simulink library "Fricciones"  (Simulink 8.3)
settings: Solver=ode45  StartTime=0.0  StopTime=10.0  RelTol=1e-3
undefined symbols (not defined in the file): Fc, Fc2, Fm, Friccion, Fs, Fs2, Fsc, mu_pts, Normal_Force_Pist_Cyl, To
libraries: nesl_utility x10, fl_lib x8, Fricciones x4, MS2G_SS_Intf_Lib x1
settings Model: Creator=Sebastian  LastModifiedBy=Sebastian

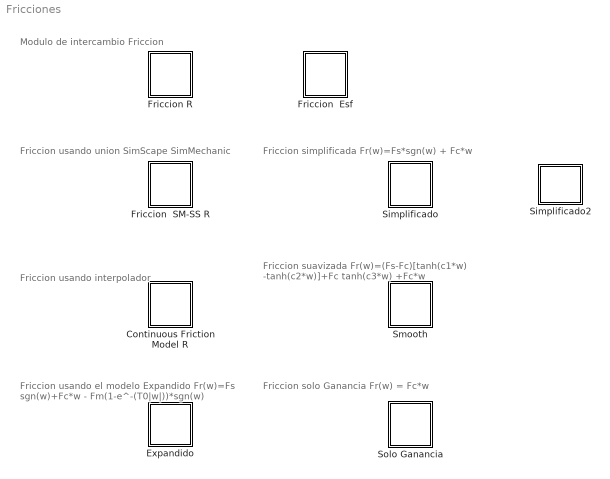
== system Fricciones ==
  note: Friccion usando
      | union SimScape
      | SimMechanic
  note: Modulo de
      | intercambio Friccion
  note: Friccion
      | simplificada
      |
      | Fr(w)=Fs*sgn(w) + Fc*w
  note: Friccion suavizada
      |
      | Fr(w)=(Fs-Fc)[tanh(c1*w)
      | -tanh(c2*w)]+Fc tanh(c3*w)
      | +Fc*w
  note: Friccion usando
      | el modelo
      | Expandido
      |
      | Fr(w)=Fs sgn(w)+Fc*w -
      | Fm(1-e^-(T0|w|))*sgn(w)
  note: Friccion solo
      | Ganancia
      |
      | Fr(w) = Fc*w
  note: Friccion usando
      | interpolador
  Continuous Friction Model R : Subsystem  mask{muk=Fc, mus=Fs, vth=0}
      mask init:
      | %%FRICTION CURVE
      | % Velocity vs. coefficient of friction
      | 
      | % NUMBER OF POINTS ON CURVE
      | num_fs_pts = 101;
      | 
      | % CURVE LIMITS
      | v_lowlim = -3*vth;
      | v_upplim = 3*vth;
      | 
      | % GENERATE X-AXIS POINTS (velocity)
      | v_pts = linspace(v_lowlim, v_upplim, num_fs_pts);
      | 
      | % DETERMINE Y-AXIS POINTS (coefficient of friction)
      | for i=1:num_fs_pts
      |     if(v_pts(i)<(-1.5*vth))
      |         mu_pts(i) = -muk;
      |     elseif(v_pts(i)>=-1.5*vth && v_pts(i)<-vth)
      |         mu_pts(i) = -(muk-mus)/(0.5*vth)*(-1.5*vth-v_pts(i))-muk;
      |     elseif(v_pts(i)>=-vth && v_pts(i)<vth)
      |         mu_pts(i) = -(mus)/vth*(-vth-v_pts(i))-mus;
      |     elseif(v_pts(i)>=vth && v_pts(i)<1.5*vth)
      |         mu_pts(i) = (muk-mus)/(0.5*vth)*(v_pts(i)-1.5*vth)+muk;
      |     elseif(v_pts(i)>=(1.5*vth))
      |         mu_pts(i) = muk;
      |     end
      | end
  Expandido : Subsystem
      mask init:
      | %To=0.1
      | %Fm=0.2
  Friccion  Esf : Subsystem
  Friccion  SM-SS R : Subsystem  mask{BFT=Fs, CFT=Fc, VFc=Fsc, Tac=5}
      mask prompts: BFT "Breakaway friction torque (N*m)"; CFT "Coulomb friction torque (N*m)"; VFc "Viscous friction coeff (N*m/(rad/s))"; Tac "Transition approximation coeff (s/rad)"
  Friccion R : Subsystem
  Simplificado : Subsystem
  Simplificado2 : Subsystem
  Smooth : Subsystem
      mask init:
      | C1=15;
      | C2=1.5;
      | C3=900;
  Solo Ganancia : Subsystem

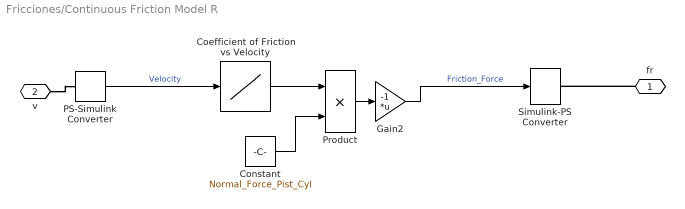
== system Fricciones/Continuous Friction Model R ==
  Coefficient of Friction vs Velocity : Lookup  InputValues=v_pts  Table=mu_pts
  Constant : Constant  Value=Normal_Force_Pist_Cyl
  Gain2 : Gain  Gain=-1  Multiplication=Matrix(K*u)  SaturateOnIntegerOverflow=on  OutDataTypeStr=Inherit: Same as input  ParamDataTypeStr=Inherit: Same as input
  PS-Simulink Converter : nesl_utility/PS-Simulink Converter  PhysicalDomain=network_engine_domain  SubClassName=ps_output  LeftPortType=input  RightPortType=output  PseudoPeriodic=off  Frequencies=[]  Unit=1  AffineConversion=off
  Product : Product  RndMeth=Zero
  Simulink-PS Converter : nesl_utility/Simulink-PS Converter  PhysicalDomain=network_engine_domain  SubClassName=ps_input  LeftPortType=input  RightPortType=output  PseudoPeriodic=off  Frequencies=[]  NoiseDistribution=none  NoiseParameters=[]  Unit=1  AffineConversion=off  InputFiltering=off  SimscapeFilterOrder=1  InputFilterTimeConstant=0.001  UdotUserProvided=1
  fr : PMIOPort  Port=1  Side=Left
  v : PMIOPort  Port=2  Side=Right
  wires:
  PS-Simulink Converter/1 -> Coefficient of Friction vs Velocity/1  "Velocity"
  Coefficient of Friction vs Velocity/1 -> Product/1
  Product/1 -> Gain2/1
  Gain2/1 -> Simulink-PS Converter/1  "Friction_Force"
  Constant/1 -> Product/2
  connections:
  v/RConn1 -- PS-Simulink Converter/LConn1
  fr/RConn1 -- Simulink-PS Converter/RConn1

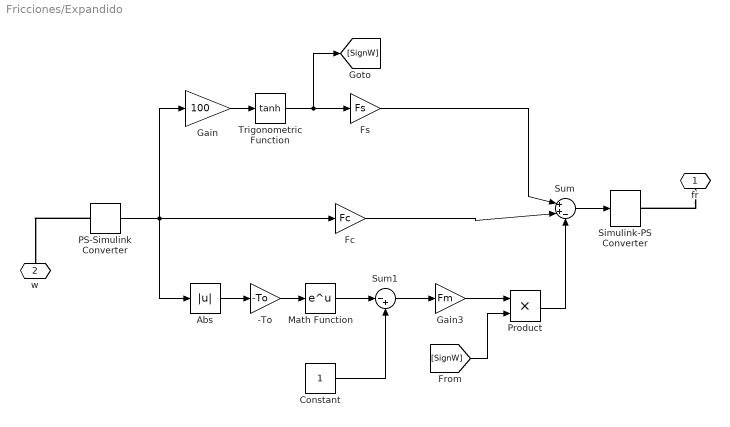
== system Fricciones/Expandido ==
  -To : Gain  Gain=-To
  Abs : Abs
  Constant : Constant
  Fc : Gain  Gain=Fc
  Fs : Gain  Gain=Fs
  Gain : Gain  Gain=100
  Gain3 : Gain  Gain=Fm
  Math Function : Math  SaturateOnIntegerOverflow=on
  PS-Simulink Converter : nesl_utility/PS-Simulink Converter  PhysicalDomain=network_engine_domain  SubClassName=ps_output  LeftPortType=input  RightPortType=output  PseudoPeriodic=off  Frequencies=[]  Unit=1  AffineConversion=off
  Product : Product
  Simulink-PS Converter : nesl_utility/Simulink-PS Converter  PhysicalDomain=network_engine_domain  SubClassName=ps_input  LeftPortType=input  RightPortType=output  PseudoPeriodic=off  Frequencies=[]  NoiseDistribution=none  NoiseParameters=[]  Unit=1  AffineConversion=off  InputFiltering=off  SimscapeFilterOrder=1  InputFilterTimeConstant=0.001  UdotUserProvided=1
  Sum : Sum  Inputs=|++-
  Sum1 : Sum  Inputs=|-+
  Trigonometric Function : Trigonometry  Operator=tanh
  fr : PMIOPort  Port=1  Side=Left
  w : PMIOPort  Port=2  Side=Right
  wires:
  Gain/1 -> Trigonometric Function/1
  Trigonometric Function/1 -> [SignW], Fs/1
  PS-Simulink Converter/1 -> Gain/1, Abs/1, Fc/1
  Fs/1 -> Sum/1
  Fc/1 -> Sum/2
  Abs/1 -> -To/1
  -To/1 -> Math Function/1
  Math Function/1 -> Sum1/1
  Constant/1 -> Sum1/2
  Sum1/1 -> Gain3/1
  Product/1 -> Sum/3
  Sum/1 -> Simulink-PS Converter/1
  Gain3/1 -> Product/1
  [SignW] -> Product/2
  connections:
  PS-Simulink Converter/LConn1 -- w/RConn1
  fr/RConn1 -- Simulink-PS Converter/RConn1

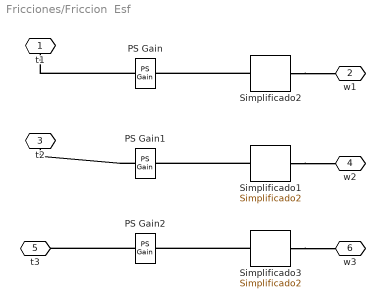
== system Fricciones/Friccion  Esf ==
  PS Gain : fl_lib/Physical Signals/Functions/PS Gain  gain=-1
  PS Gain1 : fl_lib/Physical Signals/Functions/PS Gain  gain=-1
  PS Gain2 : fl_lib/Physical Signals/Functions/PS Gain  gain=-1
  Simplificado1 : Fricciones/Simplificado2
  Simplificado2 : Fricciones/Simplificado2
  Simplificado3 : Fricciones/Simplificado2
  t1 : PMIOPort  Port=1  Side=Left
  w1 : PMIOPort  Port=2  Side=Right
  t2 : PMIOPort  Port=3  Side=Left
  w2 : PMIOPort  Port=4  Side=Right
  t3 : PMIOPort  Port=5  Side=Left
  w3 : PMIOPort  Port=6  Side=Right
  connections:
  Simplificado3/RConn1 -- w3/RConn1
  Simplificado1/RConn1 -- w2/RConn1
  Simplificado3/LConn1 -- PS Gain2/LConn1
  Simplificado1/LConn1 -- PS Gain1/LConn1
  Simplificado2/LConn1 -- PS Gain/LConn1
  Simplificado2/RConn1 -- w1/RConn1
  PS Gain2/RConn1 -- t3/RConn1
  PS Gain/RConn1 -- t1/RConn1
  PS Gain1/RConn1 -- t2/RConn1

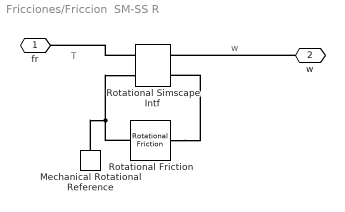
== system Fricciones/Friccion  SM-SS R ==
  note: T
  note: w
  Mechanical Rotational Reference : fl_lib/Mechanical/Rotational Elements/Mechanical Rotational Reference
  Rotational Simscape Intf : MS2G_SS_Intf_Lib/Rotational Simscape Intf
  Rotational Friction : fl_lib/Mechanical/Rotational Elements/Rotational Friction  brkwy_trq=BFT N*m  Col_trq=CFT N*m  visc_coef=VFc N*m/(rad/s)  trans_coef=Tac s/rad  vel_thr=1e-4 rad/s  w_specify=on  w_priority=High  w=0 rad/s  t_specify=on  t_priority=High  t=0 N*m
  fr : PMIOPort  Port=1  Side=Left
  w : PMIOPort  Port=2  Side=Right
  connections:
  Rotational Friction/RConn1 -- Rotational Simscape Intf/RConn2 -- Mechanical Rotational Reference/LConn1
  w/RConn1 -- Rotational Simscape Intf/LConn1
  Rotational Friction/LConn1 -- Rotational Simscape Intf/LConn2
  Rotational Simscape Intf/RConn1 -- fr/RConn1

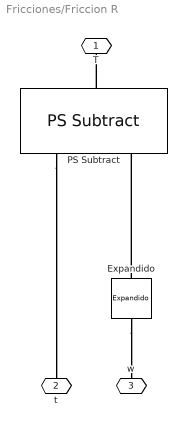
== system Fricciones/Friccion R ==
  Expandido : Fricciones/Expandido  SystemSampleTime=-1
  PS Subtract : fl_lib/Physical Signals/Functions/PS Subtract
  T : PMIOPort  Port=1  Side=Right
  t : PMIOPort  Port=2  Side=Left
  w : PMIOPort  Port=3  Side=Right
  connections:
  PS Subtract/LConn1 -- t/RConn1
  PS Subtract/RConn1 -- T/RConn1
  Expandido/RConn1 -- w/RConn1
  Expandido/LConn1 -- PS Subtract/LConn2

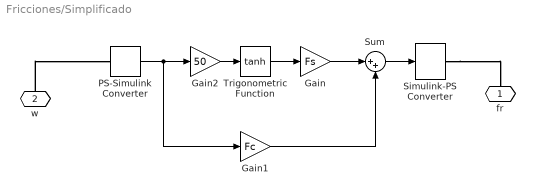
== system Fricciones/Simplificado ==
  Gain : Gain  Gain=Fs
  Gain1 : Gain  Gain=Fc
  Gain2 : Gain  Gain=50
  PS-Simulink Converter : nesl_utility/PS-Simulink Converter  PhysicalDomain=network_engine_domain  SubClassName=ps_output  LeftPortType=input  RightPortType=output  PseudoPeriodic=off  Frequencies=[]  Unit=1  AffineConversion=off
  Simulink-PS Converter : nesl_utility/Simulink-PS Converter  PhysicalDomain=network_engine_domain  SubClassName=ps_input  LeftPortType=input  RightPortType=output  PseudoPeriodic=off  Frequencies=[]  NoiseDistribution=none  NoiseParameters=[]  Unit=1  AffineConversion=off  InputFiltering=off  SimscapeFilterOrder=1  InputFilterTimeConstant=0.001  UdotUserProvided=1
  Sum : Sum  Inputs=|++
  Trigonometric Function : Trigonometry  Operator=tanh
  fr : PMIOPort  Port=1  Side=Left
  w : PMIOPort  Port=2  Side=Right
  wires:
  Sum/1 -> Simulink-PS Converter/1
  PS-Simulink Converter/1 -> Gain2/1, Gain1/1
  Gain/1 -> Sum/1
  Gain1/1 -> Sum/2
  Gain2/1 -> Trigonometric Function/1
  Trigonometric Function/1 -> Gain/1
  connections:
  w/RConn1 -- PS-Simulink Converter/LConn1
  Simulink-PS Converter/RConn1 -- fr/RConn1

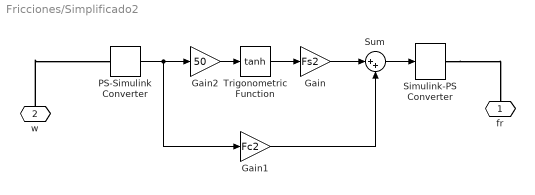
== system Fricciones/Simplificado2 ==
  Gain : Gain  Gain=Fs2
  Gain1 : Gain  Gain=Fc2
  Gain2 : Gain  Gain=50
  PS-Simulink Converter : nesl_utility/PS-Simulink Converter  PhysicalDomain=network_engine_domain  SubClassName=ps_output  LeftPortType=input  RightPortType=output  PseudoPeriodic=off  Frequencies=[]  Unit=1  AffineConversion=off
  Simulink-PS Converter : nesl_utility/Simulink-PS Converter  PhysicalDomain=network_engine_domain  SubClassName=ps_input  LeftPortType=input  RightPortType=output  PseudoPeriodic=off  Frequencies=[]  NoiseDistribution=none  NoiseParameters=[]  Unit=1  AffineConversion=off  InputFiltering=off  SimscapeFilterOrder=1  InputFilterTimeConstant=0.001  UdotUserProvided=1
  Sum : Sum  Inputs=|++
  Trigonometric Function : Trigonometry  Operator=tanh
  fr : PMIOPort  Port=1  Side=Left
  w : PMIOPort  Port=2  Side=Right
  wires:
  Gain1/1 -> Sum/2
  Gain/1 -> Sum/1
  PS-Simulink Converter/1 -> Gain2/1, Gain1/1
  Sum/1 -> Simulink-PS Converter/1
  Gain2/1 -> Trigonometric Function/1
  Trigonometric Function/1 -> Gain/1
  connections:
  Simulink-PS Converter/RConn1 -- fr/RConn1
  w/RConn1 -- PS-Simulink Converter/LConn1

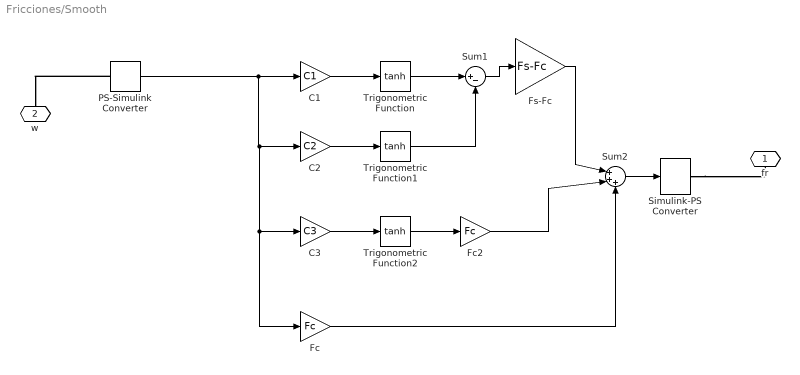
== system Fricciones/Smooth ==
  C1 : Gain  Gain=C1
  C2 : Gain  Gain=C2
  C3 : Gain  Gain=C3
  Fc : Gain  Gain=Fc
  Fc2 : Gain  Gain=Fc
  Fs-Fc : Gain  Gain=Fs-Fc
  PS-Simulink Converter : nesl_utility/PS-Simulink Converter  PhysicalDomain=network_engine_domain  SubClassName=ps_output  LeftPortType=input  RightPortType=output  PseudoPeriodic=off  Frequencies=[]  Unit=1  AffineConversion=off
  Simulink-PS Converter : nesl_utility/Simulink-PS Converter  PhysicalDomain=network_engine_domain  SubClassName=ps_input  LeftPortType=input  RightPortType=output  PseudoPeriodic=off  Frequencies=[]  NoiseDistribution=none  NoiseParameters=[]  Unit=1  AffineConversion=off  InputFiltering=off  SimscapeFilterOrder=1  InputFilterTimeConstant=0.001  UdotUserProvided=1
  Sum1 : Sum  Inputs=|+-
  Sum2 : Sum  Inputs=|+++
  Trigonometric Function : Trigonometry  Operator=tanh
  Trigonometric Function1 : Trigonometry  Operator=tanh
  Trigonometric Function2 : Trigonometry  Operator=tanh
  fr : PMIOPort  Port=1  Side=Left
  w : PMIOPort  Port=2  Side=Right
  wires:
  PS-Simulink Converter/1 -> Fc/1, C3/1, C2/1, C1/1
  Trigonometric Function/1 -> Sum1/1
  Trigonometric Function2/1 -> Fc2/1
  Sum1/1 -> Fs-Fc/1
  Trigonometric Function1/1 -> Sum1/2
  C3/1 -> Trigonometric Function2/1
  Fs-Fc/1 -> Sum2/1
  Fc2/1 -> Sum2/2
  Fc/1 -> Sum2/3
  C2/1 -> Trigonometric Function1/1
  C1/1 -> Trigonometric Function/1
  Sum2/1 -> Simulink-PS Converter/1
  connections:
  PS-Simulink Converter/LConn1 -- w/RConn1
  Simulink-PS Converter/RConn1 -- fr/RConn1

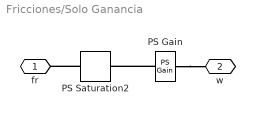
== system Fricciones/Solo Ganancia ==
  PS Gain : fl_lib/Physical Signals/Functions/PS Gain  gain=-Friccion
  PS Saturation2 : fl_lib/Physical Signals/Nonlinear Operators/PS Saturation  upper_limit=0.1  lower_limit=- 0.1
  fr : PMIOPort  Port=1  Side=Left
  w : PMIOPort  Port=2  Side=Right
  connections:
  PS Gain/RConn1 -- PS Saturation2/LConn1
  PS Saturation2/RConn1 -- fr/RConn1
  PS Gain/LConn1 -- w/RConn1
